simulink model "modelofisicocompletoo"  (R2020a)
settings: Solver=FixedStepAuto  StartTime=0.0  StopTime=inf  FixedStep=0.5e-3  MaxStep=1e-3  RelTol=1e-3
PreLoadFcn:
  | Boat_State = Simulink.Signal;
  | Boat_State.DataType = 'double';
  | Boat_State.SamplingMode = 'Sample based';
  | Boat_State.InitialValue = '[6; 5; 10; 6;  3; 4]';
  | Boat_State.StorageClass = 'ExportedGlobal';
  | Boat_State.Complexity = 'real';
  | Boat_State.Description = 'dsm_description';
undefined symbols (not defined in the file): bac, baiz, bcx, bcy, Beqtran, Bheqd, bw, DiscIntNeverNeededParam, g, Kcy, ksac, ksaiz, ksiac, ksiaiz, Kw, lh0, Meq, Mheq, Rd, Rr, rt, rtd, xl0, xt0, yl0, yt0
libraries: simulink x13, powerlib_meascontrol x4, opclib x4, vrlib x2, dspswit3 x1
(part 1 of 2)
settings Model: SimulationMode=accelerator  Creator=tomas  LastModifiedBy=lucia
settings DataIOCC: ReturnWorkspaceOutputs=off
settings OptimizationCC: EfficientMapNaN2IntZero=off
settings DebuggingCC: ArithmeticOperatorsInVariantConditions=warning
settings HardwareCC: ProdBitPerPointer=32  ProdBitPerSizeT=32  ProdBitPerPtrDiffT=32  ProdWordSize=32  ProdHWDeviceType=Intel->x86-32 (Windows32)  TargetBitPerPointer=64  TargetBitPerSizeT=64  TargetBitPerPtrDiffT=64  TargetLongLongMode=on  TargetIntDivRoundTo=Zero  TargetEndianess=LittleEndian  TargetWordSize=64  TargetHWDeviceType=MATLAB Host  ProdEqTarget=off
settings SFSimCC: SimUseLocalCustomCode=off  CustomCodeUndefinedFunction=UseInterfaceOnly
settings RTWCC: RTWUseLocalCustomCode=off
settings CodeAppCC: MaxIdLength=128  StateflowObjectComments=on
settings GRTTargetCC: TargetLangStandard=C89/C90 (ANSI)  CombineOutputUpdateFcns=off  GRTInterface=on
settings SimscapeCC: SimscapeNormalizeSystem=off
settings ConfigComp: PLC_TargetIDE=codesys35  PLC_ExternalDefinedNames=Boat_State Load_state Stable_FW_flag Total_mass Automatic_mode container_x_position  PLC_GenerateReport=off

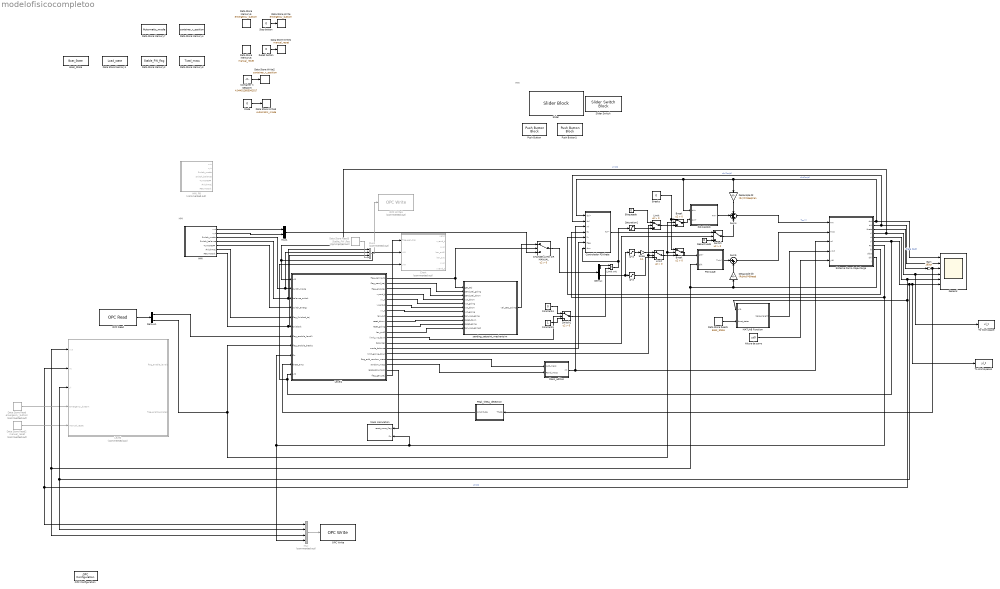
== system modelofisicocompletoo ==
  note: HMI
  note: HMI
  0/-3 : Saturate  UpperLimit=0.0  LowerLimit=-3.0
  3/-3 : Saturate  UpperLimit=3.0  LowerLimit=-3.0
  Altura de carro : Constant  Value=yt0
  Bloqueado : Constant  Value=0
  Boat_State : DataStoreMemory  DataStoreName=Boat_State  ReadBeforeWriteMsg=warning  WriteAfterWriteMsg=warning  WriteAfterReadMsg=warning  InitialValue=[5;5;6;4;8;6]  ShowAdditionalParam=off  OutDataTypeStr=double
      settings: RTWStateStorageClass=ExportedGlobal
  Break : Switch  Criteria=u2 > Threshold
  "Break " : Switch  Criteria=u2 > Threshold
  Breaks : Constant  Value=0
  CHANGE AUTO OR MANUAL : Switch  Criteria=u2 > Threshold
  Chart : Stateflow chart  Commented=on  TreatAsAtomicUnit=on
  Constant3 : Constant
  Constant4 : Constant  Value=0
  Container X Setpoint : Constant  Value=4.044012605042017  OutDataTypeStr=int8
  Controlador PD theta : Subsystem
  Data Store Memory1 : DataStoreMemory  DataStoreName=Load_state  ReadBeforeWriteMsg=warning  WriteAfterWriteMsg=warning  WriteAfterReadMsg=warning  ShowAdditionalParam=off  OutDataTypeStr=int8
      settings: RTWStateStorageClass=ExportedGlobal
  Data Store Memory2 : DataStoreMemory  DataStoreName=Stable_FW_flag  ReadBeforeWriteMsg=warning  WriteAfterWriteMsg=warning  WriteAfterReadMsg=warning  ShowAdditionalParam=off  OutDataTypeStr=boolean
      settings: RTWStateStorageClass=ExportedGlobal
  Data Store Memory3 : DataStoreMemory  DataStoreName=Total_mass  ReadBeforeWriteMsg=warning  WriteAfterWriteMsg=warning  WriteAfterReadMsg=warning  InitialValue=15000.0  ShowAdditionalParam=off  OutDataTypeStr=double
      settings: RTWStateStorageClass=ExportedGlobal
  Data Store Memory4 : DataStoreMemory  DataStoreName=container_x_position  ReadBeforeWriteMsg=warning  WriteAfterWriteMsg=warning  WriteAfterReadMsg=warning  InitialValue=2.0  ShowAdditionalParam=off  OutDataTypeStr=int8
      settings: RTWStateStorageClass=ExportedGlobal
  Data Store Memory5 : DataStoreMemory  DataStoreName=emergency_buttom  ReadBeforeWriteMsg=warning  WriteAfterWriteMsg=warning  WriteAfterReadMsg=warning  ShowAdditionalParam=off
  Data Store Memory6 : DataStoreMemory  DataStoreName=manual_reset  ReadBeforeWriteMsg=warning  WriteAfterWriteMsg=warning  WriteAfterReadMsg=warning  ShowAdditionalParam=off
  Data Store Memory7 : DataStoreMemory  DataStoreName=Automatic_mode  ReadBeforeWriteMsg=warning  WriteAfterWriteMsg=warning  WriteAfterReadMsg=warning  ShowAdditionalParam=off  OutDataTypeStr=int8
      settings: RTWStateStorageClass=ExportedGlobal
  Data Store Read : DataStoreRead  Commented=on  DataStoreName=emergency_buttom
  Data Store Read1 : DataStoreRead  DataStoreName=Boat_State
  Data Store Read2 : DataStoreRead  Commented=on  DataStoreName=manual_reset
  Data Store Read3 : DataStoreRead  Commented=on  DataStoreName=Stable_FW_flag
  Data Store Write : DataStoreWrite  DataStoreName=emergency_buttom
  Data Store Write1 : DataStoreWrite  DataStoreName=manual_reset
  Data Store Write2 : DataStoreWrite  DataStoreName=container_x_position
  Data Store Write3 : DataStoreWrite  DataStoreName=Automatic_mode
  Demux : Demux  Outputs=2
  Demux1 : Demux  Outputs=2
  Desacople bh : Gain  Gain=(Rd/rtd)*Bheqd
  Desacople bt : Gain  Gain=(Rr/rt)*Beqtran
  Desactivado : Constant  Value=0
  Gain : Gain  Gain=180/pi
  General : Scope  NumInputPorts=6
  HMI : Subsystem
  HMI_P8 : Subsystem  Commented=on
  Leve0 : Stateflow chart  Commented=on  TreatAsAtomicUnit=on
  Level1 : Stateflow chart  TreatAsAtomicUnit=on
  Limit : Switch  Criteria=u2 > Threshold
  "Limit " : Switch  Criteria=u2 > Threshold
  Limit vxt : Product
  MATLAB Function : MATLAB Function  TreatAsAtomicUnit=on
  Mass calculation : Subsystem
  Mass_adition : Subsystem
  Mode : Constant  Value=0  OutDataTypeStr=int8
  Mux : Mux  Commented=on
  Mux1 : Mux  Inputs=2
  Mux2 : Mux  Commented=on
  OPC Configuration : opclib/OPC Configuration  opcServers=localhost/CoDeSys.OPC.DA/10  errMissingItems=Error  errReadWrite=Warn  errShutdown=Error  errRTViolation=Warn  rtEnable=off  speedup=10  showLatency=off  beingUsed=on
      settings: SourceProductBaseCode=OT
  OPC Read : opclib/OPC Read  serverHost=localhost  serverID=CoDeSys.OPC.DA  itemIDs=Level1.Application.GVL0.flag_enable_level1, Level1.Application.GVL0.flag_enable_brakes  readMode=Synchronous (device)  dataType=double  updateRate=0.01  showQual=off  showTS=off  tsMode=Seconds since start
      settings: SourceProductBaseCode=OT
  OPC Write : opclib/OPC Write  serverHost=localhost  serverID=CoDeSys.OPC.DA  itemIDs=Level1.Application.GVL0.xt, Level1.Application.GVL0.yl, Level1.Application.GVL0.vyt, Level1.Application.GVL0.Fw  writeMode=Synchronous  updateRate=0.01
      settings: SourceProductBaseCode=OT
  OPC Write1 : opclib/OPC Write  Commented=on  serverHost=localhost  serverID=CoDeSys.OPC.DA  itemIDs=Level1.Application.GVL0.balancer_switch, Level1.Application.GVL0.switch_mode, Level1.Application.GVL0.twistlock, Level1.Application.GVL0.Stable_FW_flag  writeMode=Synchronous  updateRate=0.01
      settings: SourceProductBaseCode=OT
  "PID CARRO " : Subsystem
  PID IZAJE : Subsystem
  Peak_theta_detection : Subsystem  TreatAsAtomicUnit=on
  Push Button : PushButtonBlock  LabelPosition=Top  ButtonText=STOP
  Push Button1 : PushButtonBlock  LabelPosition=Top  ButtonText=RESET
  Reset button : Constant  Value=0
  Saturation1 : Saturate  UpperLimit=4.0  LowerLimit=-4.0
  Scale : Gain  Gain=0.1
  "Sistema Carro-Izaje-Carga " : Subsystem
  Slider : SliderBlock  ScaleMax=6  TickInterval=1
  Slider Switch : SliderSwitchBlock
      settings: Values={{'Ciclo simple', 'Ciclo Doble'}, [0 1]}
  "Stop button " : Constant  Value=0
  Sum4 : Sum  Inputs=+++
  Sum5 : Sum  Inputs=|++
  Switch : Switch  Criteria=u2 > Threshold
  Switch1 : Switch  Criteria=u2 > Threshold
  To Workspace : ToWorkspace  VariableName=xl_t  SampleTime=-1
  To Workspace1 : ToWorkspace  VariableName=yl_t  SampleTime=-1
  sending_setpoint_mechanisim : Subsystem
  wires:
  Sum4/1 -> "Sistema Carro-Izaje-Carga "/1(Tm)  "Tm***"
  Desacople bt/1 -> Sum4/1
  Desacople bh/1 -> Sum5/2
  PID IZAJE/1("Tmh* ") -> Sum5/1
  Switch/1 -> Sum4/3
  Sum5/1 -> "Sistema Carro-Izaje-Carga "/2(Tmh)
  MATLAB Function/1(base_height) -> "Sistema Carro-Izaje-Carga "/4(ycxt)
  Altura de carro/1 -> "Sistema Carro-Izaje-Carga "/5(yt0)
  "Sistema Carro-Izaje-Carga "/1(dxt) -> Controlador PD theta/1(dxl*), "PID CARRO "/1(dxt), Desacople bt/1, General/1  "dxt [m/s]"
  "Sistema Carro-Izaje-Carga "/10(dhl) -> Mux/3, Leve0/1(vyt), PID IZAJE/2(dlh), Desacople bh/1
  Controlador PD theta/1(Tc**) -> Switch/1
  Desactivado/1 -> Switch/3
  "Sistema Carro-Izaje-Carga "/8(lh) -> Controlador PD theta/5(lh)
  "Sistema Carro-Izaje-Carga "/2(dxl) -> Controlador PD theta/2(dxl), General/2  "dxl [m/s]"
  "Sistema Carro-Izaje-Carga "/3(theta) -> Gain/1  "theta [rad]"
  "Sistema Carro-Izaje-Carga "/4(xl) -> Level1/1(xl0), Chart/2(xl0), To Workspace/1, General/4  "xl [m]"
  "Sistema Carro-Izaje-Carga "/5(xt) -> Mux/1, Leve0/2(xt), MATLAB Function/1(xl0), General/5  "xt [m]"
  "PID CARRO "/1(Tm*) -> Sum4/2
  Gain/1 -> Peak_theta_detection/1(Theta), General/3
  Level1/13(balancer) -> Switch/2
  HMI/4(Switch_balance) -> Level1/3(balance_switch), Mux2/1
  HMI/3(Switch_mode) -> Mux2/2, Level1/2(switch_mode)
  HMI/1(vxt) -> Mux1/1
  HMI/2(vyt) -> Mux1/2
  Level1/1(flag_semiauto) -> sending_setpoint_mechanisim/1(get_traj), CHANGE AUTO OR MANUAL/2
  CHANGE AUTO OR MANUAL/1 -> Demux/1
  Demux/2 -> 0/-3/1, 3/-3/1
  Peak_theta_detection/1(Amplitude) -> Level1/10(theta_amp)
  Mux1/1 -> CHANGE AUTO OR MANUAL/3
  HMI/5(TurnONOFF) -> Level1/4(switch_energy)
  HMI/6(FinishTraj) -> Level1/5(flag_finished_taj)
  HMI/7(ReturnDock) -> Mux2/3, Level1/6(twistlock)
  Level1/2(flag_send_traj) -> sending_setpoint_mechanisim/2(send_traj_going)
  Level1/3(flag_end_traj) -> sending_setpoint_mechanisim/3(send_traj_down)
  sending_setpoint_mechanisim/1(vel_sets_points) -> CHANGE AUTO OR MANUAL/1
  Level1/7(vx_t) -> sending_setpoint_mechanisim/7(vxt_going)
  Level1/5(vy_t) -> sending_setpoint_mechanisim/5(vyt_going)
  Level1/4(vyend_t) -> sending_setpoint_mechanisim/4(vyt_down)
  Level1/6(vxend_t) -> sending_setpoint_mechanisim/6(vxt_down)
  Level1/8(len_out) -> sending_setpoint_mechanisim/8(len_vec_going)
  Level1/10(reset_going) -> sending_setpoint_mechanisim/10(reset_going)
  Level1/9(reset_down) -> sending_setpoint_mechanisim/9(reset_down)
  Level1/14(mode_balance) -> Controlador PD theta/6("flag ")
  Saturation1/1 -> Limit/3
  Level1/11(len_out2) -> sending_setpoint_mechanisim/11(len_vec_going2)
  "Limit "/1 -> "Break "/3
  0/-3/1 -> Scale/1
  Limit/1 -> Break/3
  Bloqueado/1 -> Limit/1
  Scale/1 -> "Limit "/1
  3/-3/1 -> "Limit "/3
  Level1/12(limit_vxt_down) -> Switch1/2
  Constant3/1 -> Switch1/3
  Constant4/1 -> Switch1/1
  Demux/1 -> Limit vxt/1
  Switch1/1 -> Limit vxt/2
  Limit vxt/1 -> Controlador PD theta/7(dxc), Saturation1/1
  Data Store Read1/1 -> MATLAB Function/2(boat_state)
  Mass_adition/1(ml) -> "Sistema Carro-Izaje-Carga "/3(ml), Controlador PD theta/3(ml)
  Level1/16(flag_add_random_mass) -> Mass_adition/1(Add_mass)
  Level1/17(random_mass) -> Mass_adition/2(Rand_mass)
  Level1/18(reset_calc_mass) -> Mass calculation/1(reset_mass_flag)
  Break/1 -> "PID CARRO "/2(dxt*)
  "Break "/1 -> PID IZAJE/1(dlh*)
  Demux1/2 -> Level1/8(flag_enable_breaks), "Break "/2, Break/2
  Breaks/1 -> "Break "/1, Break/1
  Data Store Read/1 -> Leve0/4(emergency_buttom)
  Data Store Read2/1 -> Leve0/5(manual_reset)
  Mode/1 -> Data Store Write3/1
  "Stop button "/1 -> Data Store Write/1
  Reset button/1 -> Data Store Write1/1
  Container X Setpoint/1 -> Data Store Write2/1
  Level1/15(limit_going_down) -> Limit/2, "Limit "/2
  Mux/1 -> OPC Write/1
  OPC Read/1 -> Demux1/1
  Demux1/1 -> Level1/7(flag_enable_level1)
  Mux2/1 -> OPC Write1/1
  "Sistema Carro-Izaje-Carga "/7(Fw) -> Mux/4, Level1/9(Fw), Mass calculation/2(Fw), Controlador PD theta/4(fw)
  Data Store Read3/1 -> Mux2/4
  "Sistema Carro-Izaje-Carga "/6(yl) -> Mux/2, Leve0/3(yl), To Workspace1/1, General/6, Chart/3(yl0), Level1/11(yl0)
  Level1/19(flag_gen_traj) -> Chart/1(flag_gen_traj)

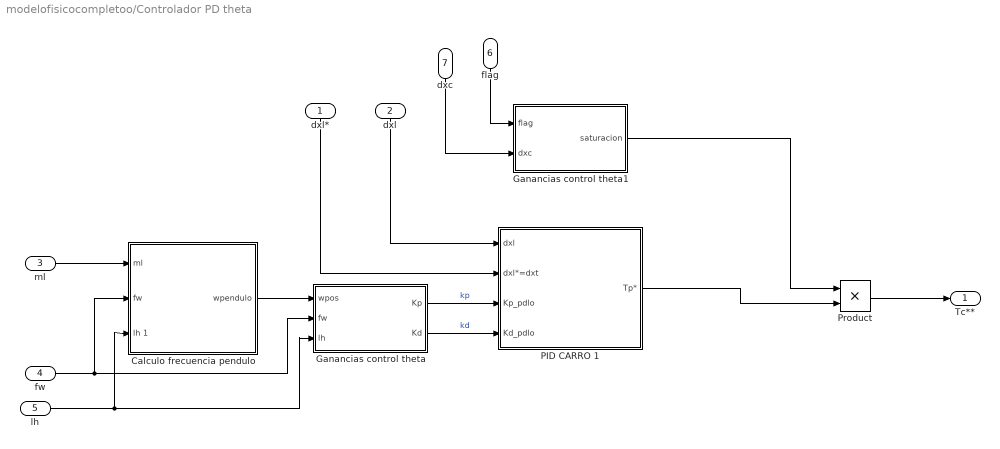
== system modelofisicocompletoo/Controlador PD theta ==
  dxl* : Inport
  dxl : Inport  Port=2
  ml : Inport  Port=3
  fw : Inport  Port=4
  lh : Inport  Port=5
  "flag " : Inport  Port=6
  dxc : Inport  Port=7
  Calculo frecuencia pendulo : Subsystem
  Ganancias control theta : MATLAB Function  TreatAsAtomicUnit=on
  Ganancias control theta1 : MATLAB Function  TreatAsAtomicUnit=on
  PID CARRO 1 : Subsystem
  Product : Product
  Tc** : Outport
  wires:
  Calculo frecuencia pendulo/1("wpendulo ") -> Ganancias control theta/1(wpos)
  ml/1 -> Calculo frecuencia pendulo/1("ml ")
  Ganancias control theta/1(Kp) -> PID CARRO 1/3(Kp_pdlo)  "kp"
  Ganancias control theta/2(Kd) -> PID CARRO 1/4(Kd_pdlo)  "kd"
  dxl/1 -> PID CARRO 1/1(dxl)
  lh/1 -> Calculo frecuencia pendulo/3(lh 1), Ganancias control theta/3(lh)
  fw/1 -> Calculo frecuencia pendulo/2("fw "), Ganancias control theta/2(fw)
  dxl*/1 -> PID CARRO 1/2(dxl*=dxt)
  PID CARRO 1/1(Tp*) -> Product/2
  dxc/1 -> Ganancias control theta1/2(dxc)
  Ganancias control theta1/1(saturacion) -> Product/1
  "flag "/1 -> Ganancias control theta1/1(flag)
  Product/1 -> Tc**/1

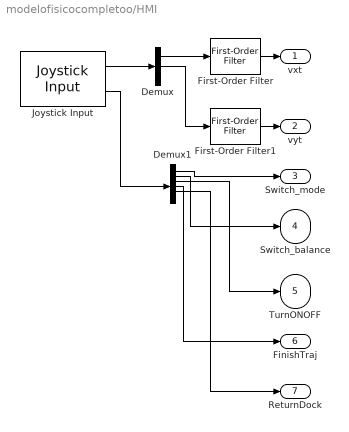
== system modelofisicocompletoo/HMI ==
  Demux : Demux  Outputs=3
  Demux1 : Demux  Outputs=6
  First-Order Filter : powerlib_meascontrol/Filters/First-Order Filter  FilterType=Lowpass  Tc=10e-3  Ts=0  Initialize=off  Vac_Init=[0, 0, 60]  Vdc_Init=0  PlotResponse=off  FreqRange="[0,  200,  1]"
  First-Order Filter1 : powerlib_meascontrol/Filters/First-Order Filter  FilterType=Lowpass  Tc=10e-3  Ts=0  Initialize=off  Vac_Init=[0, 0, 60]  Vdc_Init=0  PlotResponse=off  FreqRange="[0,  200,  1]"
  Joystick Input : vrlib/Joystick Input  joyid=1  adjustports=on  forcefeed=off
  vxt : Outport
  vyt : Outport  Port=2
  Switch_mode : Outport  Port=3
  Switch_balance : Outport  Port=4
  TurnONOFF : Outport  Port=5
  FinishTraj : Outport  Port=6
  ReturnDock : Outport  Port=7
  wires:
  First-Order Filter1/1 -> vyt/1
  First-Order Filter/1 -> vxt/1
  Demux1/2 -> Switch_balance/1
  Joystick Input/2 -> Demux1/1
  Demux1/1 -> Switch_mode/1
  Joystick Input/1 -> Demux/1
  Demux/1 -> First-Order Filter/1
  Demux/2 -> First-Order Filter1/1
  Demux1/3 -> TurnONOFF/1
  Demux1/4 -> FinishTraj/1
  Demux1/5 -> ReturnDock/1

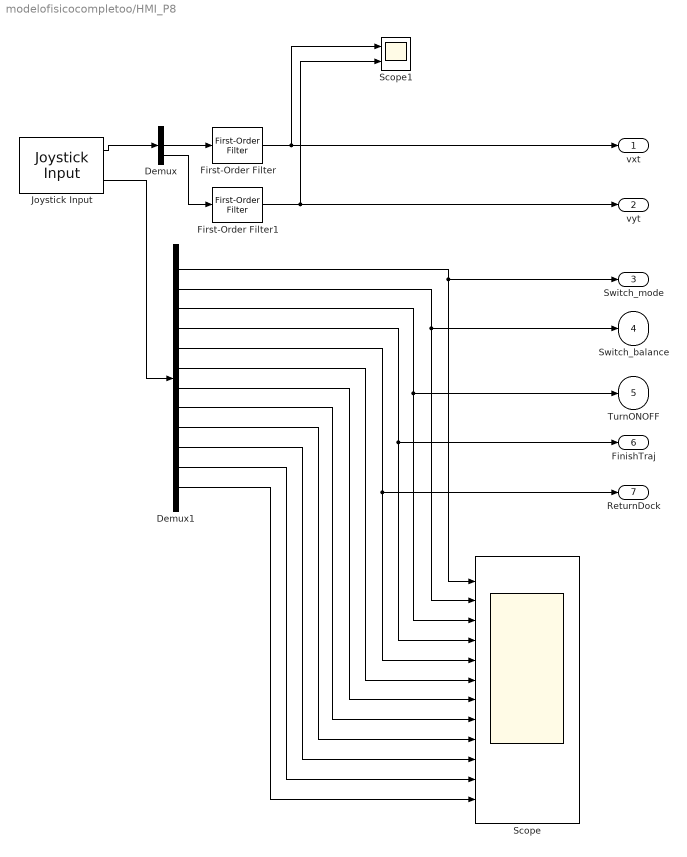
== system modelofisicocompletoo/HMI_P8 ==
  Demux : Demux  Outputs=3
  Demux1 : Demux  Outputs=12
  First-Order Filter : powerlib_meascontrol/Filters/First-Order Filter  FilterType=Lowpass  Tc=10e-3  Ts=0  Initialize=off  Vac_Init=[0, 0, 60]  Vdc_Init=0  PlotResponse=off  FreqRange="[0,  200,  1]"
  First-Order Filter1 : powerlib_meascontrol/Filters/First-Order Filter  FilterType=Lowpass  Tc=10e-3  Ts=0  Initialize=off  Vac_Init=[0, 0, 60]  Vdc_Init=0  PlotResponse=off  FreqRange="[0,  200,  1]"
  Joystick Input : vrlib/Joystick Input  joyid=1  adjustports=on  forcefeed=off
  Scope : Scope  NumInputPorts=12
  Scope1 : Scope  NumInputPorts=2
  vxt : Outport
  vyt : Outport  Port=2
  Switch_mode : Outport  Port=3
  Switch_balance : Outport  Port=4
  TurnONOFF : Outport  Port=5
  FinishTraj : Outport  Port=6
  ReturnDock : Outport  Port=7
  wires:
  Joystick Input/1 -> Demux/1
  Demux1/12 -> Scope/12
  Demux1/11 -> Scope/11
  Demux1/10 -> Scope/10
  Demux1/9 -> Scope/9
  Demux1/8 -> Scope/8
  Demux1/7 -> Scope/7
  Demux1/6 -> Scope/6
  Demux1/5 -> Scope/5, ReturnDock/1
  Demux1/4 -> Scope/4, FinishTraj/1
  Demux1/3 -> Scope/3, TurnONOFF/1
  Demux1/2 -> Scope/2, Switch_balance/1
  Demux1/1 -> Scope/1, Switch_mode/1
  Demux/3 -> First-Order Filter1/1
  Demux/2 -> First-Order Filter/1
  Joystick Input/2 -> Demux1/1
  First-Order Filter/1 -> vxt/1, Scope1/1
  First-Order Filter1/1 -> vyt/1, Scope1/2

== system modelofisicocompletoo/Mass calculation ==
  reset_mass_flag : Inport
  Fw : Inport  Port=2
  Data Store Read : DataStoreRead  DataStoreName=Load_state
  Subsystem : Subsystem
  Subsystem1 : Subsystem
  wires:
  Fw/1 -> Subsystem1/1(Fw), Subsystem/1(Fw)
  Data Store Read/1 -> Subsystem/Enable
  reset_mass_flag/1 -> Subsystem1/Enable, Subsystem/2(In1)

== system modelofisicocompletoo/Mass_adition ==
  Add_mass : Inport
  Rand_mass : Inport  Port=2
  Constant : Constant  Value=0
  Constant2 : Constant  Value=15000
  Sum1 : Sum
  add_random_mass : Switch  Criteria=u2 > Threshold
  ml : Outport
  wires:
  Add_mass/1 -> add_random_mass/2
  Constant/1 -> add_random_mass/3
  add_random_mass/1 -> Sum1/2
  Constant2/1 -> Sum1/1
  Sum1/1 -> ml/1
  Rand_mass/1 -> add_random_mass/1

== system modelofisicocompletoo/PID CARRO  ==
  dxt : Inport
  dxt* : Inport  Port=2
  Discrete-Time Integrator : DiscreteIntegrator  SampleTime=-1  ICPrevOutput=DiscIntNeverNeededParam  ICPrevScaledInput=DiscIntNeverNeededParam
  Discrete-Time Integrator1 : DiscreteIntegrator  SampleTime=-1  ICPrevOutput=DiscIntNeverNeededParam  ICPrevScaledInput=DiscIntNeverNeededParam
  Sum : Sum  Inputs=-+|
  Sum1 : Sum  Inputs=+++
  bac : Gain  Gain=bac
  ksac : Gain  Gain=ksac
  ksiac : Gain  Gain=ksiac
  Tm* : Outport
  wires:
  dxt*/1 -> Sum/2
  dxt/1 -> Sum/1
  Sum1/1 -> Tm*/1
  bac/1 -> Sum1/1
  ksac/1 -> Sum1/2
  Discrete-Time Integrator1/1 -> ksiac/1
  ksiac/1 -> Sum1/3
  Sum/1 -> Discrete-Time Integrator/1, bac/1
  Discrete-Time Integrator/1 -> Discrete-Time Integrator1/1, ksac/1

== system modelofisicocompletoo/PID IZAJE ==
  dlh* : Inport
  dlh : Inport  Port=2
  Discrete-Time Integrator1 : DiscreteIntegrator  SampleTime=-1  ICPrevOutput=DiscIntNeverNeededParam  ICPrevScaledInput=DiscIntNeverNeededParam
  Discrete-Time Integrator2 : DiscreteIntegrator  SampleTime=-1  ICPrevOutput=DiscIntNeverNeededParam  ICPrevScaledInput=DiscIntNeverNeededParam
  Sum2 : Sum  Inputs=|+-
  Sum3 : Sum  Inputs=+++
  baiz : Gain  Gain=baiz
  ksaiz : Gain  Gain=ksaiz
  ksiaiz : Gain  Gain=ksiaiz
  "Tmh* " : Outport
  wires:
  dlh/1 -> Sum2/2
  Sum3/1 -> "Tmh* "/1
  ksaiz/1 -> Sum3/2
  Discrete-Time Integrator2/1 -> ksiaiz/1
  baiz/1 -> Sum3/1
  ksiaiz/1 -> Sum3/3
  dlh*/1 -> Sum2/1
  Sum2/1 -> Discrete-Time Integrator1/1, baiz/1
  Discrete-Time Integrator1/1 -> Discrete-Time Integrator2/1, ksaiz/1

== system modelofisicocompletoo/Peak_theta_detection ==
  Theta : Inport
  Detect Decrease : simulink/Logic and Bit Operations/Detect Decrease  vinit=0.0  OutDataTypeStr=boolean
  Detect Rise Positive : simulink/Logic and Bit Operations/Detect Rise Positive  vinit=0  OutDataTypeStr=boolean
  MinMax Running Resettable : simulink/Math Operations/MinMax Running Resettable  Function=max  vinit=0.0
  Subsystem : Subsystem
  Amplitude : Outport
  wires:
  Theta/1 -> Detect Decrease/1, Detect Rise Positive/1, MinMax Running Resettable/1
  Subsystem/1(Out1) -> Amplitude/1
  MinMax Running Resettable/1 -> Subsystem/1(In1)
  Detect Rise Positive/1 -> MinMax Running Resettable/2
  Detect Decrease/1 -> Subsystem/Trigger

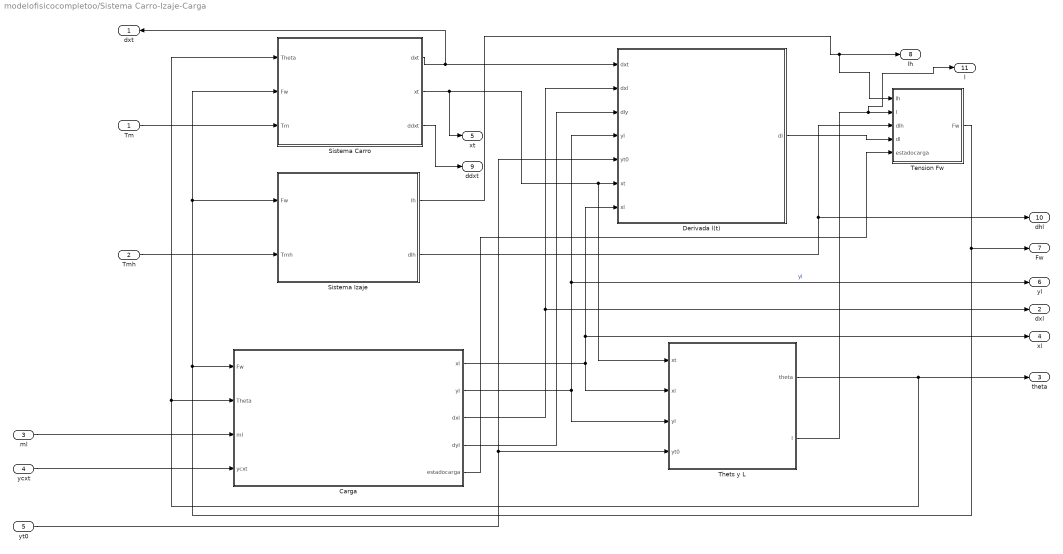
== system modelofisicocompletoo/Sistema Carro-Izaje-Carga  ==
  Tm : Inport
  Tmh : Inport  Port=2
  ml : Inport  Port=3
  ycxt : Inport  Port=4
  yt0 : Inport  Port=5
  "Carga " : Subsystem
  Derivada l(t) : Subsystem
  Sistema Carro : Subsystem
  Sistema Izaje : Subsystem
  Tension Fw : Subsystem
  Thets y L : Subsystem
  dxt : Outport
  dxl : Outport  Port=2
  theta : Outport  Port=3
  xl : Outport  Port=4
  xt : Outport  Port=5
  yl : Outport  Port=6
  Fw : Outport  Port=7
  lh : Outport  Port=8
  ddxt : Outport  Port=9
  dhl : Outport  Port=10
  l : Outport  Port=11
  wires:
  Sistema Carro/2(xt) -> xt/1, Derivada l(t)/6(xt), Thets y L/1(xt)
  Sistema Carro/1("dxt ") -> dxt/1, Derivada l(t)/1(dxt)
  Sistema Izaje/1(lh) -> Tension Fw/1(lh), lh/1
  Sistema Izaje/2(dlh) -> dhl/1, Tension Fw/3(dlh)
  "Carga "/2(yl) -> yl/1, Derivada l(t)/4(yl), Thets y L/3(yl)  "yl"
  "Carga "/3(dxl) -> dxl/1, Derivada l(t)/2(dxl)
  "Carga "/4(dyl) -> Derivada l(t)/3(dly)
  Derivada l(t)/1(dl) -> Tension Fw/4(dl)
  Thets y L/1("theta ") -> theta/1, Sistema Carro/1(Theta), "Carga "/2(Theta)
  ml/1 -> "Carga "/3(ml)
  ycxt/1 -> "Carga "/4(ycxt)
  "Carga "/5("estadocarga ") -> Tension Fw/5(estadocarga)
  Thets y L/2("l ") -> l/1, Tension Fw/2(l)
  Tm/1 -> Sistema Carro/3(Tm)
  Tmh/1 -> Sistema Izaje/2(Tmh)
  yt0/1 -> Derivada l(t)/5(yt0), Thets y L/4(yt0)
  "Carga "/1(xl) -> Derivada l(t)/7(xl), xl/1, Thets y L/2(xl)
  Tension Fw/1("Fw ") -> Fw/1, Sistema Carro/2(Fw), Sistema Izaje/1(Fw), "Carga "/1(Fw)
  Sistema Carro/3("ddxt ") -> ddxt/1

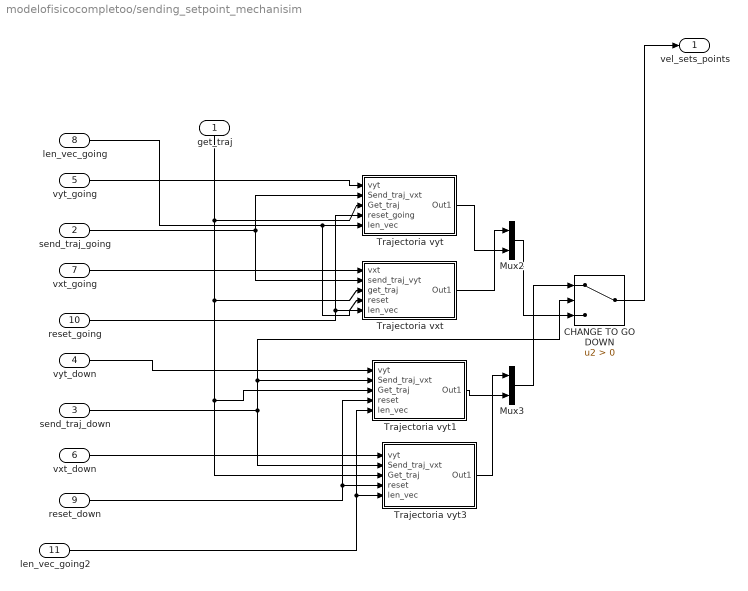
== system modelofisicocompletoo/sending_setpoint_mechanisim ==
  get_traj : Inport
  send_traj_going : Inport  Port=2
  send_traj_down : Inport  Port=3
  vyt_down : Inport  Port=4
  vyt_going : Inport  Port=5
  vxt_down : Inport  Port=6
  vxt_going : Inport  Port=7
  len_vec_going : Inport  Port=8
  reset_down : Inport  Port=9
  reset_going : Inport  Port=10
  len_vec_going2 : Inport  Port=11
  CHANGE TO GO DOWN : Switch  Criteria=u2 > Threshold
  Mux2 : Mux  Inputs=2
  Mux3 : Mux  Inputs=2
  Trajectoria vxt : Subsystem
  Trajectoria vyt : Subsystem
  Trajectoria vyt1 : Subsystem
  Trajectoria vyt3 : Subsystem
  vel_sets_points : Outport
  wires:
  get_traj/1 -> Trajectoria vyt3/3(Get_traj), Trajectoria vyt1/3(Get_traj), Trajectoria vxt/3("get_traj "), Trajectoria vyt/3(Get_traj)
  vyt_going/1 -> Trajectoria vyt/1("vyt ")
  Trajectoria vxt/1(Out1) -> Mux2/1
  Trajectoria vyt/1(Out1) -> Mux2/2
  vxt_going/1 -> Trajectoria vxt/1(vxt)
  send_traj_going/1 -> Trajectoria vxt/2(send_traj_vyt), Trajectoria vyt/2("Send_traj_vxt ")
  vyt_down/1 -> Trajectoria vyt1/1("vyt ")
  vxt_down/1 -> Trajectoria vyt3/1("vyt ")
  send_traj_down/1 -> Trajectoria vyt3/2("Send_traj_vxt "), Trajectoria vyt1/2("Send_traj_vxt "), CHANGE TO GO DOWN/2
  Trajectoria vyt1/1(Out1) -> Mux3/2
  Trajectoria vyt3/1(Out1) -> Mux3/1
  CHANGE TO GO DOWN/1 -> vel_sets_points/1
  Mux3/1 -> CHANGE TO GO DOWN/1
  Mux2/1 -> CHANGE TO GO DOWN/3
  reset_going/1 -> Trajectoria vxt/4(reset), Trajectoria vyt/4(reset_going)
  reset_down/1 -> Trajectoria vyt3/4(reset), Trajectoria vyt1/4(reset)
  len_vec_going/1 -> Trajectoria vxt/5(len_vec), Trajectoria vyt/5(len_vec)
  len_vec_going2/1 -> Trajectoria vyt3/5(len_vec), Trajectoria vyt1/5(len_vec)

== system modelofisicocompletoo/Controlador PD theta/Calculo frecuencia pendulo ==
  "ml " : Inport
  "fw " : Inport  Port=2
  lh 1 : Inport  Port=3
  Abs : Abs
  Divide : Product  Inputs=*/
  Gain : Gain  Gain=90
  Product : Product
  Sqrt : Sqrt  OutputSignalType=complex  SaturateOnIntegerOverflow=on
  "wpendulo " : Outport
  wires:
  "fw "/1 -> Divide/1
  Divide/1 -> Sqrt/1
  lh 1/1 -> Product/2
  Product/1 -> Divide/2
  Sqrt/1 -> Abs/1
  "ml "/1 -> Product/1
  Abs/1 -> Gain/1
  Gain/1 -> "wpendulo "/1

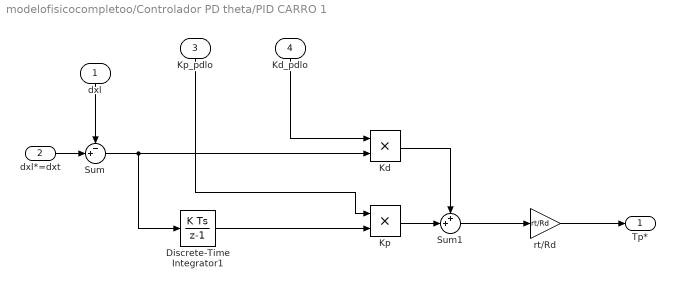
== system modelofisicocompletoo/Controlador PD theta/PID CARRO 1 ==
  dxl : Inport
  dxl*=dxt : Inport  Port=2
  Kp_pdlo : Inport  Port=3
  Kd_pdlo : Inport  Port=4
  Discrete-Time Integrator1 : DiscreteIntegrator  SampleTime=-1  ICPrevOutput=DiscIntNeverNeededParam  ICPrevScaledInput=DiscIntNeverNeededParam
  Kd : Product
  Kp : Product
  Sum : Sum  Inputs=-+|
  Sum1 : Sum  Inputs=++|
  rt/Rd : Gain  Gain=rt/Rd
  Tp* : Outport
  wires:
  dxl*=dxt/1 -> Sum/2
  dxl/1 -> Sum/1
  Sum1/1 -> rt/Rd/1
  Sum/1 -> Discrete-Time Integrator1/1, Kd/2
  Kd/1 -> Sum1/1
  Discrete-Time Integrator1/1 -> Kp/2
  Kp/1 -> Sum1/2
  Kp_pdlo/1 -> Kp/1
  Kd_pdlo/1 -> Kd/1
  rt/Rd/1 -> Tp*/1

== system modelofisicocompletoo/Mass calculation/Subsystem ==
  Fw : Inport
  In1 : Inport  Port=2
  Enable : EnablePort  StatesWhenEnabling=reset
  Data Store Write : DataStoreWrite  DataStoreName=Stable_FW_flag
  Data Store Write1 : DataStoreWrite  DataStoreName=Total_mass
  Gain : Gain  Gain=1/9.81
  Subsystem : Subsystem
  wires:
  Fw/1 -> Subsystem/1(Fw)
  Subsystem/1(Mass) -> Gain/1
  Subsystem/2(Stable_Fw_flag) -> Data Store Write/1
  In1/1 -> Subsystem/Reset
  Gain/1 -> Data Store Write1/1

== system modelofisicocompletoo/Mass calculation/Subsystem1 ==
  Fw : Inport
  Enable : EnablePort
  Data Store Write : DataStoreWrite  DataStoreName=Stable_FW_flag
  Peak_theta_detection1 : Subsystem
  wires:
  Fw/1 -> Peak_theta_detection1/1(Fw)
  Peak_theta_detection1/1(Logical_output) -> Data Store Write/1

== system modelofisicocompletoo/Peak_theta_detection/Subsystem ==
  In1 : Inport
  Trigger : TriggerPort  VariantControl=Variant  PortDimensions=1
  Out1 : Outport
  wires:
  In1/1 -> Out1/1

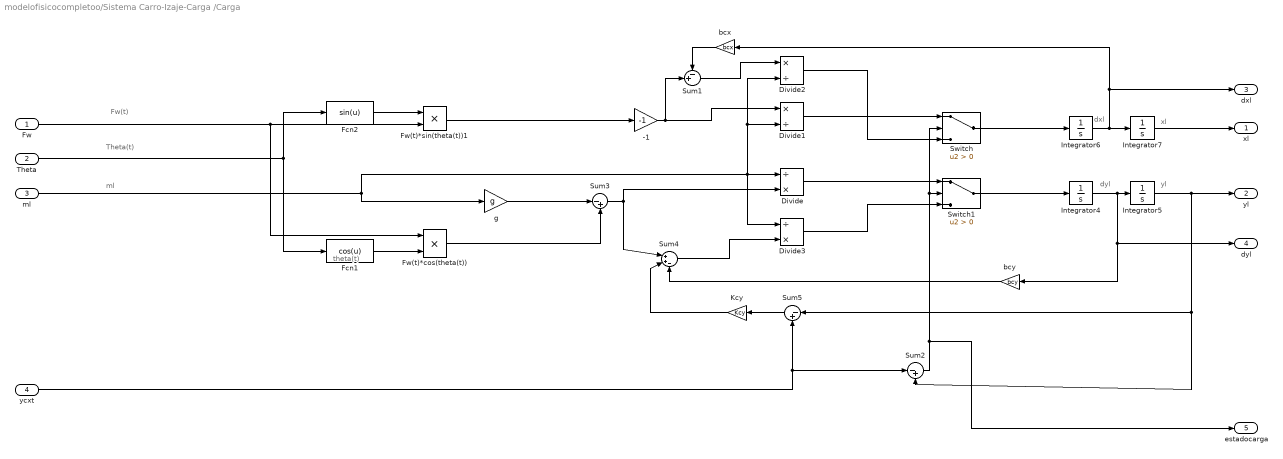
== system modelofisicocompletoo/Sistema Carro-Izaje-Carga /Carga  ==
  note: Theta(t)
  note: Fw(t)
  note: ml
  note: theta(t)
  note: dyl
  note: yl
  note: dxl
  note: xl
  Fw : Inport
  Theta : Inport  Port=2
  ml : Inport  Port=3
  ycxt : Inport  Port=4
  -1 : Gain  Gain=-1
  Divide : Product  Inputs=/*
  Divide1 : Product  Inputs=*/
  Divide2 : Product  Inputs=*/
  Divide3 : Product  Inputs=/*
  Fcn1 : Fcn  Expr=cos(u)
  Fcn2 : Fcn  Expr=sin(u)
  Fw(t)*cos(theta(t)) : Product
  Fw(t)*sin(theta(t))1 : Product
  Integrator4 : Integrator
  Integrator5 : Integrator  InitialCondition=yl0
  Integrator6 : Integrator
  Integrator7 : Integrator  InitialCondition=xl0
  Kcy : Gain  Gain=Kcy
  Sum1 : Sum  Inputs=-+|
  Sum2 : Sum  Inputs=|-+
  Sum3 : Sum  Inputs=|-+
  Sum4 : Sum  Inputs=|++-
  Sum5 : Sum  Inputs=|-+
  Switch : Switch  Criteria=u2 > Threshold
  Switch1 : Switch  Criteria=u2 > Threshold
  bcx : Gain  Gain=bcx
  bcy : Gain  Gain=bcy
  g : Gain  Gain=g
  xl : Outport
  yl : Outport  Port=2
  dxl : Outport  Port=3
  dyl : Outport  Port=4
  "estadocarga " : Outport  Port=5
  wires:
  Fcn2/1 -> Fw(t)*sin(theta(t))1/1
  Theta/1 -> Fcn1/1, Fcn2/1
  g/1 -> Sum3/1
  Fcn1/1 -> Fw(t)*cos(theta(t))/2
  Fw(t)*cos(theta(t))/1 -> Sum3/2
  Fw/1 -> Fw(t)*cos(theta(t))/1, Fw(t)*sin(theta(t))1/2
  ml/1 -> Divide1/2, Divide2/2, Divide3/1, Divide/1, g/1
  Integrator7/1 -> xl/1
  Integrator6/1 -> Integrator7/1, dxl/1, bcx/1
  Fw(t)*sin(theta(t))1/1 -> -1/1
  Integrator5/1 -> Sum2/2, Sum5/1, yl/1
  Divide1/1 -> Switch/1
  -1/1 -> Sum1/2, Divide1/1
  Integrator4/1 -> dyl/1, bcy/1, Integrator5/1
  Sum3/1 -> Sum4/1, Divide/2
  Switch/1 -> Integrator6/1
  bcx/1 -> Sum1/1
  Sum2/1 -> "estadocarga "/1, Switch1/2, Switch/2
  ycxt/1 -> Sum2/1, Sum5/2
  Sum1/1 -> Divide2/1
  Divide2/1 -> Switch/3
  Sum4/1 -> Divide3/2
  Divide3/1 -> Switch1/3
  Switch1/1 -> Integrator4/1
  Divide/1 -> Switch1/1
  Sum5/1 -> Kcy/1
  Kcy/1 -> Sum4/2
  bcy/1 -> Sum4/3

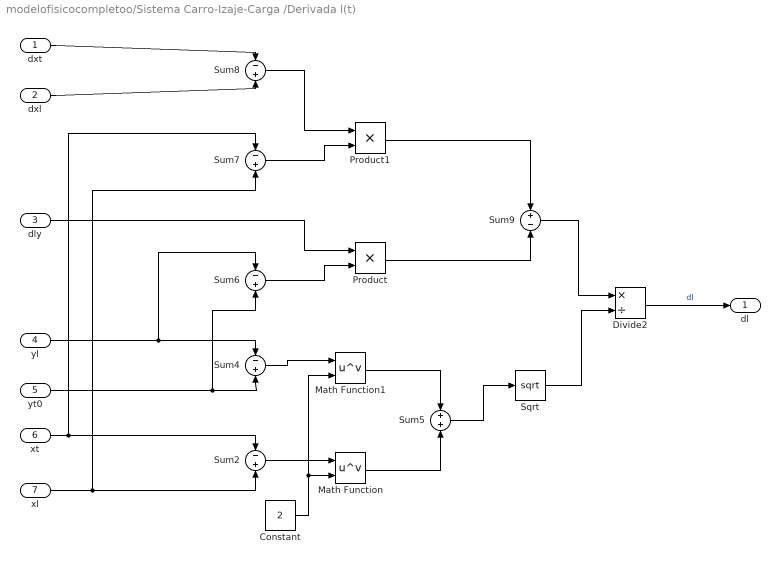
== system modelofisicocompletoo/Sistema Carro-Izaje-Carga /Derivada l(t) ==
  dxt : Inport
  dxl : Inport  Port=2
  dly : Inport  Port=3
  yl : Inport  Port=4
  yt0 : Inport  Port=5
  xt : Inport  Port=6
  xl : Inport  Port=7
  Constant : Constant  Value=2
  Divide2 : Product  Inputs=*/
  Math Function : Math  Operator=pow  SignedPower=on  SaturateOnIntegerOverflow=on
  Math Function1 : Math  Operator=pow  SignedPower=on  SaturateOnIntegerOverflow=on
  Product : Product
  Product1 : Product
  Sqrt : Sqrt  SaturateOnIntegerOverflow=on
  Sum{2,4,6..8} (5 alike) : Sum  Inputs=-+
  Sum5 : Sum
  Sum9 : Sum  Inputs=+-
  dl : Outport
  wires:
  Divide2/1 -> dl/1  "dl"
  dly/1 -> Product/1
  yl/1 -> Sum6/1, Sum4/1
  xl/1 -> Sum7/2, Sum2/2
  Product/1 -> Sum9/2
  dxt/1 -> Sum8/1
  Sum5/1 -> Sqrt/1
  Constant/1 -> Math Function1/2, Math Function/2
  yt0/1 -> Sum4/2, Sum6/2
  dxl/1 -> Sum8/2
  Math Function1/1 -> Sum5/1
  Sum8/1 -> Product1/1
  Sum9/1 -> Divide2/1
  Math Function/1 -> Sum5/2
  xt/1 -> Sum7/1, Sum2/1
  Sum6/1 -> Product/2
  Sum7/1 -> Product1/2
  Product1/1 -> Sum9/1
  Sum4/1 -> Math Function1/1
  Sqrt/1 -> Divide2/2
  Sum2/1 -> Math Function/1

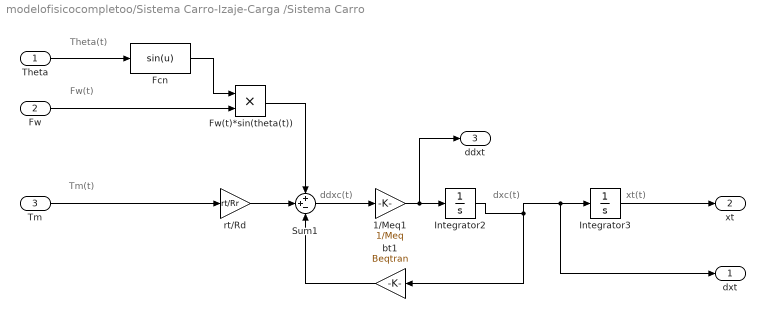
== system modelofisicocompletoo/Sistema Carro-Izaje-Carga /Sistema Carro ==
  note: dxc(t)
  note: xt(t)
  note: ddxc(t)
  note: Theta(t)
  note: Fw(t)
  note: Tm(t)
  Theta : Inport
  Fw : Inport  Port=2
  Tm : Inport  Port=3
  1/Meq1 : Gain  Gain=1/Meq
  Fcn : Fcn  Expr=sin(u)
  Fw(t)*sin(theta(t)) : Product
  Integrator2 : Integrator
  Integrator3 : Integrator  InitialCondition=xt0
  Sum1 : Sum  Inputs=++-
  bt1 : Gain  Gain=Beqtran
  rt/Rd : Gain  Gain=rt/Rr
  "dxt " : Outport
  xt : Outport  Port=2
  "ddxt " : Outport  Port=3
  wires:
  Integrator3/1 -> xt/1
  Sum1/1 -> 1/Meq1/1
  Fw/1 -> Fw(t)*sin(theta(t))/2
  Fcn/1 -> Fw(t)*sin(theta(t))/1
  rt/Rd/1 -> Sum1/2
  Theta/1 -> Fcn/1
  Fw(t)*sin(theta(t))/1 -> Sum1/1
  1/Meq1/1 -> "ddxt "/1, Integrator2/1
  Tm/1 -> rt/Rd/1
  bt1/1 -> Sum1/3
  Integrator2/1 -> "dxt "/1, Integrator3/1, bt1/1

== system modelofisicocompletoo/Sistema Carro-Izaje-Carga /Sistema Izaje ==
  note: lh(t)
  note: dlh(t)
  note: ddlh(t)
  note: Tmh(t)
  note: Fw(t)
  Fw : Inport
  Tmh : Inport  Port=2
  1/Meq : Gain  Gain=1/Mheq
  Integrator : Integrator
  Integrator1 : Integrator  InitialCondition=lh0
  Sum : Sum  Inputs=++-
  bt : Gain  Gain=Bheqd
  rtd/Rd : Gain  Gain=-rtd/Rd
  lh : Outport
  dlh : Outport  Port=2
  wires:
  Integrator/1 -> dlh/1, bt/1, Integrator1/1
  Integrator1/1 -> lh/1
  rtd/Rd/1 -> Sum/2
  bt/1 -> Sum/3
  Fw/1 -> Sum/1
  Tmh/1 -> rtd/Rd/1
  1/Meq/1 -> Integrator/1
  Sum/1 -> 1/Meq/1

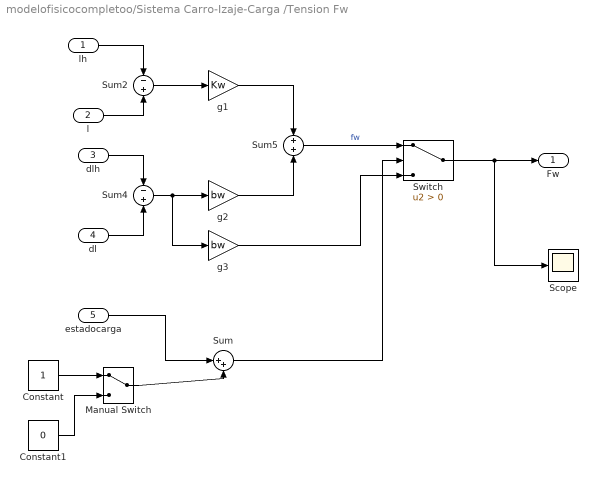
== system modelofisicocompletoo/Sistema Carro-Izaje-Carga /Tension Fw ==
  lh : Inport
  l : Inport  Port=2
  dlh : Inport  Port=3
  dl : Inport  Port=4
  estadocarga : Inport  Port=5
  Constant : Constant
  Constant1 : Constant  Value=0
  Manual Switch : ManualSwitch
  Scope : Scope
  Sum : Sum  Inputs=|++
  Sum2 : Sum  Inputs=-+
  Sum4 : Sum  Inputs=-+
  Sum5 : Sum
  Switch : Switch  Criteria=u2 > Threshold
  g1 : Gain  Gain=Kw
  g2 : Gain  Gain=bw
  g3 : Gain  Gain=bw
  "Fw " : Outport
  wires:
  l/1 -> Sum2/2
  dl/1 -> Sum4/2
  g2/1 -> Sum5/2
  Sum5/1 -> Switch/1  "fw"
  Sum4/1 -> g3/1, g2/1
  g1/1 -> Sum5/1
  dlh/1 -> Sum4/1
  g3/1 -> Switch/3
  lh/1 -> Sum2/1
  Switch/1 -> Scope/1, "Fw "/1
  Sum2/1 -> g1/1
  Constant/1 -> Manual Switch/1
  Constant1/1 -> Manual Switch/2
  Manual Switch/1 -> Sum/2
  estadocarga/1 -> Sum/1
  Sum/1 -> Switch/2

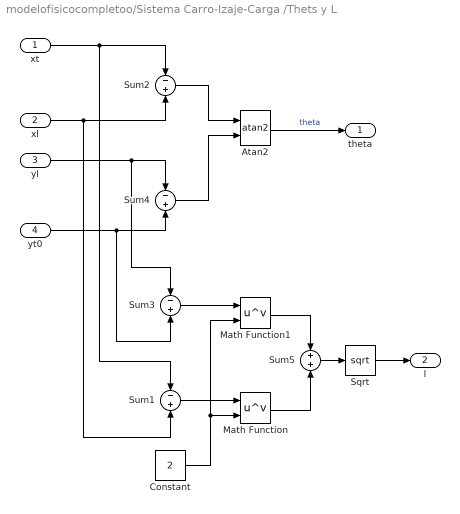
== system modelofisicocompletoo/Sistema Carro-Izaje-Carga /Thets y L ==
  xt : Inport
  xl : Inport  Port=2
  yl : Inport  Port=3
  yt0 : Inport  Port=4
  Atan2 : Trigonometry  Operator=atan2
  Constant : Constant  Value=2
  Math Function : Math  Operator=pow  SignedPower=on  SaturateOnIntegerOverflow=on
  Math Function1 : Math  Operator=pow  SignedPower=on  SaturateOnIntegerOverflow=on
  Sqrt : Sqrt  SaturateOnIntegerOverflow=on
  Sum{1..4} (4 alike) : Sum  Inputs=-+
  Sum5 : Sum
  "theta " : Outport
  "l " : Outport  Port=2
  wires:
  Sum4/1 -> Atan2/2
  xt/1 -> Sum1/1, Sum2/1
  xl/1 -> Sum1/2, Sum2/2
  yt0/1 -> Sum3/2, Sum4/2
  Atan2/1 -> "theta "/1  "theta"
  yl/1 -> Sum3/1, Sum4/1
  Sum2/1 -> Atan2/1
  Sqrt/1 -> "l "/1
  Math Function/1 -> Sum5/2
  Math Function1/1 -> Sum5/1
  Sum3/1 -> Math Function1/1
  Sum1/1 -> Math Function/1
  Constant/1 -> Math Function/2, Math Function1/2
  Sum5/1 -> Sqrt/1

== system modelofisicocompletoo/sending_setpoint_mechanisim/Trajectoria vxt ==
  vxt : Inport
  send_traj_vyt : Inport  Port=2
  "get_traj " : Inport  Port=3
  reset : Inport  Port=4
  len_vec : Inport  Port=5
  Subsystem2 : Subsystem
  Subsystem3 : Subsystem
  Out1 : Outport
  wires:
  vxt/1 -> Subsystem2/1(In1)
  Subsystem2/1(Out1) -> Subsystem3/1(In1)
  send_traj_vyt/1 -> Subsystem3/Enable
  Subsystem3/1(Out1) -> Out1/1
  "get_traj "/1 -> Subsystem2/Enable
  reset/1 -> Subsystem3/2(In2)
  len_vec/1 -> Subsystem3/3(In3)

== system modelofisicocompletoo/sending_setpoint_mechanisim/Trajectoria vyt ==
  "vyt " : Inport
  "Send_traj_vxt " : Inport  Port=2
  Get_traj : Inport  Port=3
  reset_going : Inport  Port=4
  len_vec : Inport  Port=5
  Subsystem2 : Subsystem
  Subsystem3 : Subsystem
  Out1 : Outport
  wires:
  "vyt "/1 -> Subsystem2/1(In1)
  Subsystem2/1(Out1) -> Subsystem3/1(In1)
  "Send_traj_vxt "/1 -> Subsystem3/Enable
  Subsystem3/1(Out1) -> Out1/1
  Get_traj/1 -> Subsystem2/Enable
  reset_going/1 -> Subsystem3/2(In2)
  len_vec/1 -> Subsystem3/3(In3)

== system modelofisicocompletoo/sending_setpoint_mechanisim/Trajectoria vyt1 ==
  "vyt " : Inport
  "Send_traj_vxt " : Inport  Port=2
  Get_traj : Inport  Port=3
  reset : Inport  Port=4
  len_vec : Inport  Port=5
  Subsystem2 : Subsystem
  Subsystem3 : Subsystem
  Out1 : Outport
  wires:
  "vyt "/1 -> Subsystem2/1(In1)
  Subsystem2/1(Out1) -> Subsystem3/1(In1)
  "Send_traj_vxt "/1 -> Subsystem3/Enable
  Subsystem3/1(Out1) -> Out1/1
  Get_traj/1 -> Subsystem2/Enable
  reset/1 -> Subsystem3/2(In2)
  len_vec/1 -> Subsystem3/3(In3)

== system modelofisicocompletoo/sending_setpoint_mechanisim/Trajectoria vyt3 ==
  "vyt " : Inport
  "Send_traj_vxt " : Inport  Port=2
  Get_traj : Inport  Port=3
  reset : Inport  Port=4
  len_vec : Inport  Port=5
  Subsystem2 : Subsystem
  Subsystem3 : Subsystem
  Out1 : Outport
  wires:
  "vyt "/1 -> Subsystem2/1(In1)
  Subsystem2/1(Out1) -> Subsystem3/1(In1)
  "Send_traj_vxt "/1 -> Subsystem3/Enable
  Subsystem3/1(Out1) -> Out1/1
  Get_traj/1 -> Subsystem2/Enable
  reset/1 -> Subsystem3/2(In2)
  len_vec/1 -> Subsystem3/3(In3)

== system modelofisicocompletoo/Mass calculation/Subsystem/Subsystem ==
  Fw : Inport
  Reset : ResetPort  DisableCoverage=on  ResetTriggerType=either
  Gain : Gain  Gain=1/9.81
  Peak_theta_detection1 : Subsystem
  Mass : Outport
  Stable_Fw_flag : Outport  Port=2
  wires:
  Gain/1 -> Mass/1
  Fw/1 -> Peak_theta_detection1/1(Fw)
  Peak_theta_detection1/1(Amplitude) -> Gain/1
  Peak_theta_detection1/2(Logical_output) -> Stable_Fw_flag/1

== system modelofisicocompletoo/Mass calculation/Subsystem1/Peak_theta_detection1 ==
  Fw : Inport
  Compare To Constant : simulink/Logic and Bit Operations/Compare To Constant  relop=>=  const=14000*9.8  OutDataTypeStr=boolean
  Detect Decrease : simulink/Logic and Bit Operations/Detect Decrease  vinit=0.0  OutDataTypeStr=boolean
  Detect Increase : simulink/Logic and Bit Operations/Detect Increase  vinit=0.0  OutDataTypeStr=boolean
  Detect Rise Positive : simulink/Logic and Bit Operations/Detect Rise Positive  vinit=0  OutDataTypeStr=boolean
  Logical Operator : Logic  AllPortsSameDT=off  OutDataTypeStr=boolean
  MinMax Running Resettable : simulink/Math Operations/MinMax Running Resettable  Function=max  vinit=0.0
  Scope : Scope
  Subsystem : Subsystem
  Logical_output : Outport
  wires:
  Fw/1 -> Detect Decrease/1, Detect Rise Positive/1, MinMax Running Resettable/1
  MinMax Running Resettable/1 -> Subsystem/1(In1)
  Detect Rise Positive/1 -> MinMax Running Resettable/2
  Detect Decrease/1 -> Subsystem/Trigger
  Detect Increase/1 -> Logical Operator/1
  Subsystem/1(Out1) -> Scope/1, Compare To Constant/1, Detect Increase/1
  Logical Operator/1 -> Logical_output/1
  Compare To Constant/1 -> Logical Operator/2

== system modelofisicocompletoo/sending_setpoint_mechanisim/Trajectoria vxt/Subsystem2 ==
  In1 : Inport
  Enable : EnablePort
  Out1 : Outport
  wires:
  In1/1 -> Out1/1

== system modelofisicocompletoo/sending_setpoint_mechanisim/Trajectoria vxt/Subsystem3 ==
  In1 : Inport
  In2 : Inport  Port=2
  In3 : Inport  Port=3
  Enable : EnablePort
  Resettable Subsystem : Subsystem  TreatAsAtomicUnit=on
  Out1 : Outport
  wires:
  In1/1 -> Resettable Subsystem/1(In1)
  In2/1 -> Resettable Subsystem/Reset
  Resettable Subsystem/1(Out1) -> Out1/1
  In3/1 -> Resettable Subsystem/2(len_vector)

== system modelofisicocompletoo/sending_setpoint_mechanisim/Trajectoria vyt/Subsystem2 ==
  In1 : Inport
  Enable : EnablePort
  Out1 : Outport
  wires:
  In1/1 -> Out1/1

== system modelofisicocompletoo/sending_setpoint_mechanisim/Trajectoria vyt/Subsystem3 ==
  In1 : Inport
  In2 : Inport  Port=2
  In3 : Inport  Port=3
  Enable : EnablePort
  Resettable Subsystem : Subsystem  TreatAsAtomicUnit=on
  Out1 : Outport
  wires:
  In1/1 -> Resettable Subsystem/1(In1)
  In2/1 -> Resettable Subsystem/Reset
  Resettable Subsystem/1(Out1) -> Out1/1
  In3/1 -> Resettable Subsystem/2(len_vector)

== system modelofisicocompletoo/sending_setpoint_mechanisim/Trajectoria vyt1/Subsystem2 ==
  In1 : Inport
  Enable : EnablePort
  Out1 : Outport
  wires:
  In1/1 -> Out1/1

== system modelofisicocompletoo/sending_setpoint_mechanisim/Trajectoria vyt1/Subsystem3 ==
  In1 : Inport
  In2 : Inport  Port=2
  In3 : Inport  Port=3
  Enable : EnablePort
  Resettable Subsystem : Subsystem  TreatAsAtomicUnit=on
  Out1 : Outport
  wires:
  In1/1 -> Resettable Subsystem/1(In1)
  In2/1 -> Resettable Subsystem/Reset
  Resettable Subsystem/1(Out1) -> Out1/1
  In3/1 -> Resettable Subsystem/2(len_vector)

== system modelofisicocompletoo/sending_setpoint_mechanisim/Trajectoria vyt3/Subsystem2 ==
  In1 : Inport
  Enable : EnablePort
  Out1 : Outport
  wires:
  In1/1 -> Out1/1

== system modelofisicocompletoo/sending_setpoint_mechanisim/Trajectoria vyt3/Subsystem3 ==
  In1 : Inport
  In2 : Inport  Port=2
  In3 : Inport  Port=3
  Enable : EnablePort
  Resettable Subsystem : Subsystem  TreatAsAtomicUnit=on
  Out1 : Outport
  wires:
  In1/1 -> Resettable Subsystem/1(In1)
  In2/1 -> Resettable Subsystem/Reset
  Resettable Subsystem/1(Out1) -> Out1/1
  In3/1 -> Resettable Subsystem/2(len_vector)

== system modelofisicocompletoo/Mass calculation/Subsystem/Subsystem/Peak_theta_detection1 ==
  Fw : Inport
  Compare To Constant1 : simulink/Logic and Bit Operations/Compare To Constant  relop=>=  const=2  OutDataTypeStr=boolean
  Counter : dspswit3/Counter  Direction=Up  CountEvent=Rising edge  CounterSize=8 bits  MaxCount=2  InitialCount=0  Output=Count  HitValue=32  ResetInput=off  SamplesPerFrame=1  Ts=1  CntDtype=double  HitDtype=Logical
  Detect Decrease : simulink/Logic and Bit Operations/Detect Decrease  vinit=0.0  OutDataTypeStr=boolean
  Detect Increase : simulink/Logic and Bit Operations/Detect Increase  vinit=0.0  OutDataTypeStr=boolean
  Detect Rise Positive : simulink/Logic and Bit Operations/Detect Rise Positive  vinit=0  OutDataTypeStr=boolean
  MinMax Running Resettable : simulink/Math Operations/MinMax Running Resettable  Function=max  vinit=0.0
  Subsystem : Subsystem
  Amplitude : Outport
  Logical_output : Outport  Port=2
  wires:
  Fw/1 -> Detect Decrease/1, Detect Rise Positive/1, MinMax Running Resettable/1
  MinMax Running Resettable/1 -> Subsystem/1(In1)
  Detect Rise Positive/1 -> MinMax Running Resettable/2
  Detect Decrease/1 -> Subsystem/Trigger
  Detect Increase/1 -> Counter/1
  Subsystem/1(Out1) -> Amplitude/1, Detect Increase/1
  Compare To Constant1/1 -> Logical_output/1
  Counter/1 -> Compare To Constant1/1

== system modelofisicocompletoo/Mass calculation/Subsystem1/Peak_theta_detection1/Subsystem ==
  In1 : Inport
  Trigger : TriggerPort  VariantControl=Variant  PortDimensions=1
  Out1 : Outport
  wires:
  In1/1 -> Out1/1

== system modelofisicocompletoo/sending_setpoint_mechanisim/Trajectoria vxt/Subsystem3/Resettable Subsystem ==
  In1 : Inport
  len_vector : Inport  Port=2
  Reset : ResetPort  DisableCoverage=on  ResetTriggerType=either
  MATLAB Function : MATLAB Function  TreatAsAtomicUnit=on
  Memory : Memory
  Scope : Scope
  Out1 : Outport
  wires:
  len_vector/1 -> MATLAB Function/1(len_vec)
  MATLAB Function/2(vt) -> Out1/1
  MATLAB Function/1(cont) -> Scope/1, Memory/1
  Memory/1 -> MATLAB Function/3(cont_i)
  In1/1 -> MATLAB Function/2(qd)

== system modelofisicocompletoo/sending_setpoint_mechanisim/Trajectoria vyt/Subsystem3/Resettable Subsystem ==
  In1 : Inport
  len_vector : Inport  Port=2
  Reset : ResetPort  DisableCoverage=on  ResetTriggerType=either
  MATLAB Function : MATLAB Function  TreatAsAtomicUnit=on
  Memory : Memory
  Out1 : Outport
  wires:
  In1/1 -> MATLAB Function/2(qd)
  MATLAB Function/2(vt) -> Out1/1
  Memory/1 -> MATLAB Function/3(cont_i)
  MATLAB Function/1(cont) -> Memory/1
  len_vector/1 -> MATLAB Function/1(len_vec)

== system modelofisicocompletoo/sending_setpoint_mechanisim/Trajectoria vyt1/Subsystem3/Resettable Subsystem ==
  In1 : Inport
  len_vector : Inport  Port=2
  Reset : ResetPort  DisableCoverage=on  ResetTriggerType=either
  MATLAB Function : MATLAB Function  TreatAsAtomicUnit=on
  Memory : Memory
  Out1 : Outport
  wires:
  len_vector/1 -> MATLAB Function/1(len_vec)
  MATLAB Function/2(vt) -> Out1/1
  MATLAB Function/1(cont) -> Memory/1
  Memory/1 -> MATLAB Function/3(cont_i)
  In1/1 -> MATLAB Function/2(qd)

== system modelofisicocompletoo/sending_setpoint_mechanisim/Trajectoria vyt3/Subsystem3/Resettable Subsystem ==
  In1 : Inport
  len_vector : Inport  Port=2
  Reset : ResetPort  DisableCoverage=on  ResetTriggerType=either
  MATLAB Function : MATLAB Function  TreatAsAtomicUnit=on
  Memory : Memory
  Out1 : Outport
  wires:
  len_vector/1 -> MATLAB Function/1(len_vec)
  MATLAB Function/2(vt) -> Out1/1
  MATLAB Function/1(cont) -> Memory/1
  Memory/1 -> MATLAB Function/3(cont_i)
  In1/1 -> MATLAB Function/2(qd)

== system modelofisicocompletoo/Mass calculation/Subsystem/Subsystem/Peak_theta_detection1/Subsystem ==
  In1 : Inport
  Trigger : TriggerPort  VariantControl=Variant  PortDimensions=1
  Out1 : Outport
  wires:
  In1/1 -> Out1/1

== matlab function modelofisicocompletoo/MATLAB Function ==
  data: xl0 input; base_height output; boat_state input
function base_height    = get_base_height(xl0,boat_state)

boat_wide = 6;
boat_under_water = 10;
hy_cont = 2.5;


x_positions = [1.42,4.06,6.7,9.34,11.98,14.62];

if(xl0>=0)
posx_init_index = 1;
for i=1:boat_wide
    if(abs(xl0 - x_positions(i)) <= (2.44/2) + 0.1)
        posx_init_index = i;
    end
end

base_height=boat_state(posx_init_index)*hy_cont - boat_under_water;
else
base_height = hy_cont;  
posx_init_index=0;
end

end

== stateflow chart modelofisicocompletoo/Leve0 ==
  state SystemStatusOkey
    entry: flag_enable_level1 = true;
    flag_enable_brakes= 0;
  state SystemStatusEmergency
    entry: flag_enable_level1 = false;
    flag_enable_brakes= 1;
    during: flag_enable_brakes= 1;
  SystemStatusEmergency -> SystemStatusOkey : [manual_reset==1]
  SystemStatusOkey -> SystemStatusEmergency [order 1] : [xt<-40 ||  xt>60 || yl>45]
  (default) -> SystemStatusOkey
  SystemStatusOkey -> SystemStatusEmergency [order 2] : [emergency_buttom==1]
  data: flag_enable_level1 output; flag_enable_brakes output; vyt input; xt input; yl input; emergency_buttom input; manual_reset input

== stateflow chart modelofisicocompletoo/Chart ==
  state Traj_generator
    state on
      entry:  [vyt,vxt,xend,vx_end,vy_end,len,len2,nx_state] = gen_traj_boat(Boat_State,xl0,yl0,container_x_position,Load_state,Total_mass);
      vx_t=vxt; vy_t=vyt;vxend_t=vx_end;vyend_t=vy_end;len_out=len;len_out2 = len2;Boat_State=nx_state;
    state off
    (default) -> off
    on -> off : [~flag_gen_traj]
    off -> on : [flag_gen_traj]
  (default) -> Traj_generator
  data: estado_barco function_input; posx_init function_input; posy_init function_input; posx_end function_input; twistlocks function_input; vdyt function_output; vdxt function_output; x_end function_output; vxt_end function_output; vyt_end function_output; ml function_input; lenght function_output; lenght2 function_output; next_state function_output; flag_gen_traj input; xl0 input; yl0 input; xend output; vyend_t output size=20000000,1; vy_t output size=20000000,1; len_out2 output; len_out output; vx_t output size=20000000,1; vxend_t output size=20000000,1; Boat_State data_store_memory; vyt local size=20000000,1; len local; vy_end local size=20000000,1; vx_end local size=20000000,1; len2 local; nx_state local; vxt local size=20000000,1; container_x_position data_store_memory; Total_mass data_store_memory; Load_state data_store_memory
  function [vdyt,vdxt,x_end,vxt_end,vyt_end,lenght,lenght2,next_state] = gen_traj_boat(estado_barco,posx_init,posy_init,posx_end,twistlocks,ml):
    | function [vdyt,vdxt,x_end,vxt_end,vyt_end,lenght,lenght2,next_state] = gen_traj_boat(estado_barco,posx_init,posy_init,posx_end,twistlocks,ml)
    | coder.extrinsic('gen_traj_to_boat');
    | vdyt = [];
    | vdxt = [];
    | vxt_end =[];
    | vyt_end = [];
    | next_state = [0; 0; 0; 0; 0; 0];
    | x_end=0;
    | lenght=0;
    | lenght2=0;
    | coder.varsize('vdyt', [20000000 1]);
    | coder.varsize('vdxt', [20000000 1]);
    | coder.varsize('vyt_end', [20000000 1]);
    | coder.varsize('vxt_end', [20000000 1]);
    | [vdyt,vdxt,x_end,vxt_end,vyt_end,lenght,lenght2,next_state]=gen_traj_to_boat(estado_barco,posx_init,posy_init,posx_end,twistlocks, ml);
    | end

== matlab function modelofisicocompletoo/Controlador PD theta/Ganancias control theta1 ==
  data: flag input; dxc input; saturacion output
function saturacion  = fcn(flag,dxc)
    if(flag)
    if(abs(dxc)>0)
        saturacion =  1.0;
%     elseif(abs(dxc)>0.0001 && (ddxc==0))
%         saturacion =  0.7;
    else
        saturacion = 1.0;
    end
    else
    if(abs(dxc)>0)
        saturacion =  0.1;
%     elseif(abs(dxc)>0.0001 && (ddxc==0))
%         saturacion =  0.7;
    else
        saturacion = 0.1;
    end
    end
end

== matlab function modelofisicocompletoo/Controlador PD theta/Ganancias control theta ==
  data: wpos input; Kp output; Kd output; fw input; lh input
function [Kp,Kd] = fcn(wpos,fw,lh)
    Meq=59008;
    Kp=wpos^2 + (fw/(Meq*lh));
    Kd=2*wpos;
end
